simulink library "INT_AirHt_Ctl"  (R2016b)
settings: Solver=VariableStepAuto  StartTime=0.0  StopTime=10.0  RelTol=1e-3
settings Model: Creator=guanxiaoxing  LastModifiedBy=guanxiaoxing

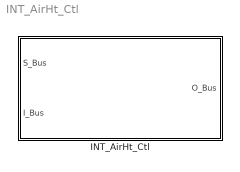
== system INT_AirHt_Ctl ==
  INT_AirHt_Ctl : Subsystem

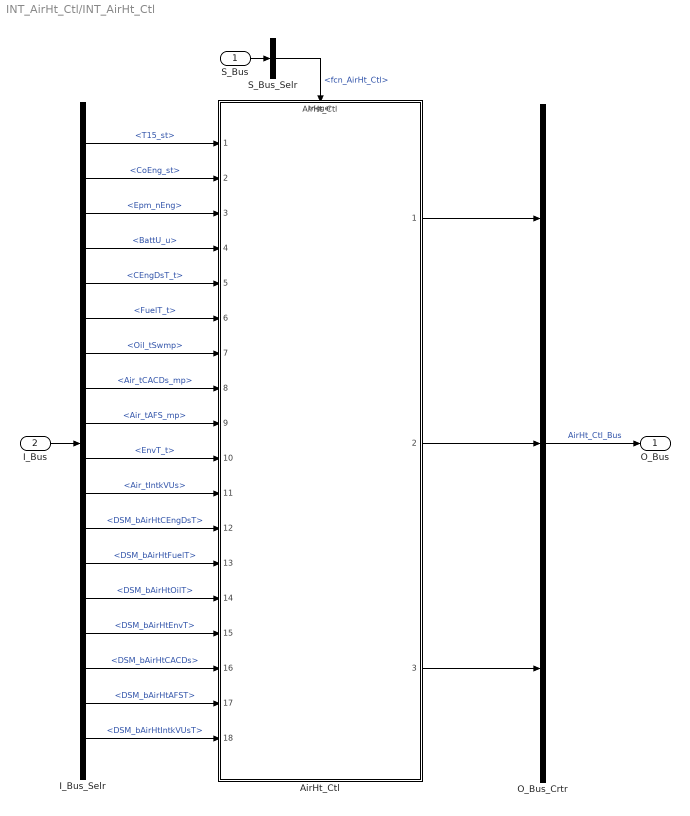
== system INT_AirHt_Ctl/INT_AirHt_Ctl ==
  S_Bus : Inport
  I_Bus : Inport  Port=2
  AirHt_Ctl : ModelReference  ModelNameDialog=AirHt_Ctl  SimulationMode=Normal  ModelReferenceVersion=1.148  TriggerPortName=function  TriggerPortTriggerType=function-call  TriggerPortStatesWhenEnabling=held
  I_Bus_Selr : BusSelector  OutputSignals=T15_st,CoEng_st,Epm_nEng,BattU_u,CEngDsT_t,FuelT_t,Oil_tSwmp,Air_tCACDs_mp,Air_tAFS_mp,EnvT_t,Air_tIntkVUs,DSM_bAirHtCEngDsT,DSM_bAirHtFuelT,DSM_bAirHtOilT,DSM_bAirHtEnvT,DSM_bAirHtCACDs,DSM_bAirHtAFST,DSM_bAirHtIntkVUsT
  O_Bus_Crtr : BusCreator  Inputs=3
  S_Bus_Selr : BusSelector  OutputSignals=fcn_AirHt_Ctl
  O_Bus : Outport
  wires:
  S_Bus_Selr/1 -> AirHt_Ctl/Trigger  "<fcn_AirHt_Ctl>"
  S_Bus/1 -> S_Bus_Selr/1
  I_Bus/1 -> I_Bus_Selr/1
  I_Bus_Selr/1 -> AirHt_Ctl/1  "<T15_st>"
  I_Bus_Selr/2 -> AirHt_Ctl/2  "<CoEng_st>"
  I_Bus_Selr/3 -> AirHt_Ctl/3  "<Epm_nEng>"
  I_Bus_Selr/4 -> AirHt_Ctl/4  "<BattU_u>"
  I_Bus_Selr/5 -> AirHt_Ctl/5  "<CEngDsT_t>"
  I_Bus_Selr/6 -> AirHt_Ctl/6  "<FuelT_t>"
  I_Bus_Selr/7 -> AirHt_Ctl/7  "<Oil_tSwmp>"
  I_Bus_Selr/8 -> AirHt_Ctl/8  "<Air_tCACDs_mp>"
  I_Bus_Selr/9 -> AirHt_Ctl/9  "<Air_tAFS_mp>"
  I_Bus_Selr/10 -> AirHt_Ctl/10  "<EnvT_t>"
  I_Bus_Selr/11 -> AirHt_Ctl/11  "<Air_tIntkVUs>"
  I_Bus_Selr/12 -> AirHt_Ctl/12  "<DSM_bAirHtCEngDsT>"
  I_Bus_Selr/13 -> AirHt_Ctl/13  "<DSM_bAirHtFuelT>"
  I_Bus_Selr/14 -> AirHt_Ctl/14  "<DSM_bAirHtOilT>"
  I_Bus_Selr/15 -> AirHt_Ctl/15  "<DSM_bAirHtEnvT>"
  I_Bus_Selr/16 -> AirHt_Ctl/16  "<DSM_bAirHtCACDs>"
  I_Bus_Selr/17 -> AirHt_Ctl/17  "<DSM_bAirHtAFST>"
  I_Bus_Selr/18 -> AirHt_Ctl/18  "<DSM_bAirHtIntkVUsT>"
  O_Bus_Crtr/1 -> O_Bus/1  "AirHt_Ctl_Bus"
  AirHt_Ctl/1 -> O_Bus_Crtr/1
  AirHt_Ctl/2 -> O_Bus_Crtr/2
  AirHt_Ctl/3 -> O_Bus_Crtr/3
